simulink model "ExampleWater"  (R2024a)
settings: Solver=FixedStepAuto  StartTime=0.0  StopTime=inf  FixedStep=0.02  RelTol=1e-3  EnableMultiTasking=on
undefined symbols (not defined in the file): atmosphericScattering, basicProperties, bloomBrightnessThreshold, bloomStrength, color, cosInnerCutOffAngle, cosOuterCutOffAngle, direction, emissionColorMultiplier, invRadiusPow4, meshID, pointLightID, position, quadraticFalloff, quaternion, reflectionColorMultiplier, refractionColorMultiplier, scale, shadowBiasMax, shadowBiasMin, shininess, specularColor, spotLightID, strengthDuDvNormal1, strengthDuDvNormal2, textureCoordinateAnimation1, textureCoordinateAnimation2, textureCoordinateScaling1, textureCoordinateScaling2, updateMesh, visible
libraries: PRISMA x49, GenericTarget x2, simulink_extras x1
settings Model: Creator=damerius  LastModifiedBy=Scythe
settings SolverCC: ConcurrentTasks=on  AlgebraicLoopSolver=TrustRegion  PositivePriorityOrder=on
settings DataIOCC: SaveOutput=off  SignalLogging=off  DSMLogging=off  SaveTime=off  ReturnWorkspaceOutputs=off
settings OptimizationCC: DefaultParameterBehavior=Inlined  ReuseModelBlockBuffer=off  ZeroExternalMemoryAtStartup=off  ZeroInternalMemoryAtStartup=off  SimCompilerOptimization=on
settings DebuggingCC: UnconnectedInputMsg=warning  UnconnectedOutputMsg=warning  UnconnectedLineMsg=warning
settings HardwareCC: ProdBitPerLong=64  ProdHWDeviceType=Intel->x86-64 (Linux 64)
settings ModelReferenceCC: EnableRefExpFcnMdlSchedulingChecks=on
settings SFSimCC: SimParseCustomCode=off  SimGenImportedTypeDefs=on  SimTargetLang=C++
settings RTWCC: GenCodeOnly=on  PackageGeneratedCodeAndArtifacts=on  PackageName=PackNGo  RTWVerbose=off  BuildConfiguration=Faster Runs  TargetLang=C++  GPUComputeCapability=3.5  DLArmComputeVersion=19.05
settings CodeAppCC: ForceParamTrailComments=on  MaxIdLength=95  MATLABSourceComments=on  UseSimReservedNames=on
settings GRTTargetCC: TargetLangStandard=C++11 (ISO)  GenerateFullHeader=off  MatFileLogging=off  CodeInterfacePackaging=C++ class

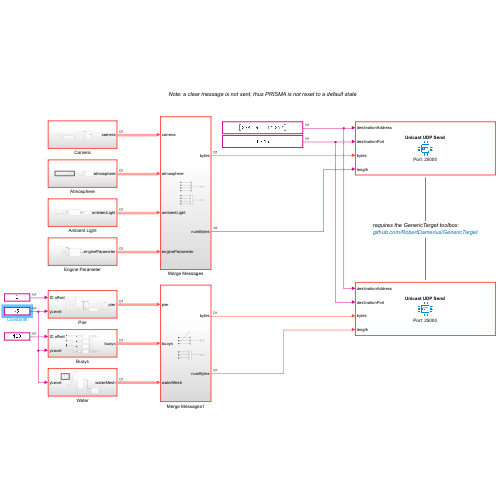
[thumbnail: Simulink's stored preview of the top-level diagram]
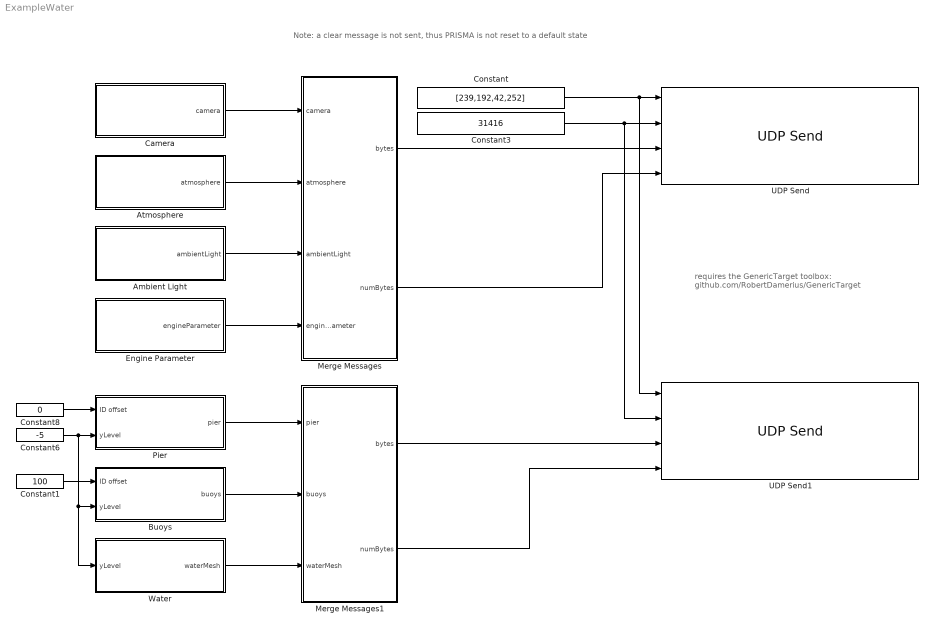
== system ExampleWater ==
  note: Note: a clear message is not sent, thus PRISMA is not reset to a default state
  note: requires the GenericTarget toolbox:
      | github.com/RobertDamerius/GenericTarget
  Ambient Light : Subsystem
  Atmosphere : Subsystem
  Buoys : Subsystem
  Camera : Subsystem
  Constant : Constant  Value=[239,192,42,252]  OutDataTypeStr=uint8
  Constant1 : Constant  Value=100  OutDataTypeStr=uint32
  Constant3 : Constant  Value=31416  OutDataTypeStr=uint16
  Constant6 : Constant  Value=-5
  Constant8 : Constant  Value=0  OutDataTypeStr=uint32
  Engine Parameter : Subsystem
  Merge Messages : Subsystem
  Merge Messages1 : Subsystem
  Pier : Subsystem
  UDP Send : GenericTarget/Interface/UDP Send  showDetails=off  interfacePort=25000  interfaceIP=[0,0,0,0]  deviceName=''  prioritySocket=6  allowBroadcast=off  SampleTime=-1
      settings: SourceProductName=Generic Target
  UDP Send1 : GenericTarget/Interface/UDP Send  showDetails=off  interfacePort=25000  interfaceIP=[0,0,0,0]  deviceName=''  prioritySocket=6  allowBroadcast=off  SampleTime=-1
      settings: SourceProductName=Generic Target
  Water : Subsystem
  wires:
  Constant3/1 -> UDP Send1/2, UDP Send/2
  Camera/1(camera) -> Merge Messages/1(camera)
  Merge Messages/1(bytes) -> UDP Send/3
  Merge Messages/2(numBytes) -> UDP Send/4
  Ambient Light/1(ambientLight) -> Merge Messages/3(ambientLight)
  Constant/1 -> UDP Send1/1, UDP Send/1
  Atmosphere/1(atmosphere) -> Merge Messages/2(atmosphere)
  Engine Parameter/1(engineParameter) -> Merge Messages/4(engineParameter)
  Constant8/1 -> Pier/1(ID offset)
  Constant1/1 -> Buoys/1(ID offset)
  Constant6/1 -> Water/1(yLevel), Buoys/2(yLevel), Pier/2(yLevel)
  Pier/1(pier) -> Merge Messages1/1(pier)
  Buoys/1(buoys) -> Merge Messages1/2(buoys)
  Water/1(waterMesh) -> Merge Messages1/3(waterMesh)
  Merge Messages1/1(bytes) -> UDP Send1/3
  Merge Messages1/2(numBytes) -> UDP Send1/4

== system ExampleWater/Ambient Light ==
  Bus Assignment2 : BusAssignment  AssignedSignals=color
  Constant12 : Constant  Value=[1;1;1]
  Default Ambient Light Bus : PRISMA/Default Ambient Light Bus
      settings: SourceProductName=PRISMA
  Gain : Gain  Gain=0.02
  Pack Ambient Light Message : PRISMA/Pack Ambient Light Message
      settings: SourceProductName=PRISMA
  Bus Element Out : Outport  PortName=ambientLight  Element=bytes
  Bus Element Out1 : Outport  PortName=ambientLight  Element=numBytes
  wires:
  Pack Ambient Light Message/2 -> Bus Element Out1/1
  Pack Ambient Light Message/1 -> Bus Element Out/1
  Gain/1 -> Bus Assignment2/2
  Constant12/1 -> Gain/1
  Default Ambient Light Bus/1 -> Bus Assignment2/1
  Bus Assignment2/1 -> Pack Ambient Light Message/1

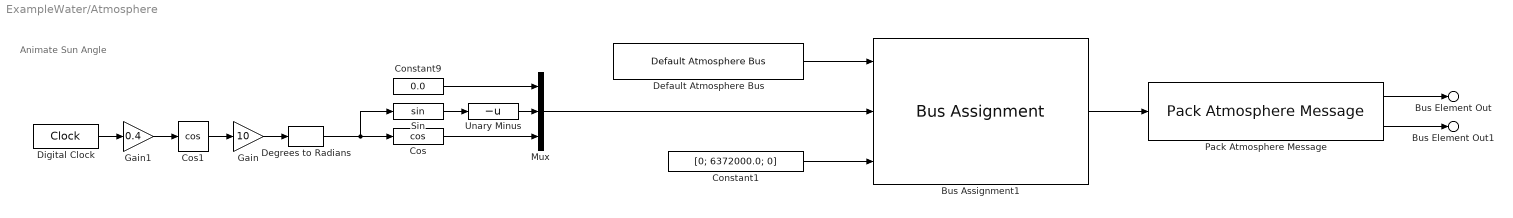
== system ExampleWater/Atmosphere ==
  note: Animate Sun Angle
  Bus Assignment1 : BusAssignment  AssignedSignals=basicProperties.sunLightDirection,atmosphericScattering.eyePosition
  Constant1 : Constant  Value=[0; 6372000.0; 0]
  Constant9 : Constant  Value=0.0
  Cos : Trigonometry  Operator=cos
  Cos1 : Trigonometry  Operator=cos
  Default Atmosphere Bus : PRISMA/Default Atmosphere Bus
      settings: SourceProductName=PRISMA
  Degrees to Radians : simulink_extras/Transformations/Degrees to Radians
  Digital Clock : DigitalClock  SampleTime=0.02
  Gain : Gain  Gain=10
  Gain1 : Gain  Gain=0.4
  Mux : Mux  Inputs=3
  Pack Atmosphere Message : PRISMA/Pack Atmosphere Message
      settings: SourceProductName=PRISMA
  Sin : Trigonometry
  Unary Minus : UnaryMinus
  Bus Element Out : Outport  PortName=atmosphere  Element=bytes
  Bus Element Out1 : Outport  PortName=atmosphere  Element=numBytes
  wires:
  Bus Assignment1/1 -> Pack Atmosphere Message/1
  Default Atmosphere Bus/1 -> Bus Assignment1/1
  Pack Atmosphere Message/1 -> Bus Element Out/1
  Pack Atmosphere Message/2 -> Bus Element Out1/1
  Mux/1 -> Bus Assignment1/2
  Constant1/1 -> Bus Assignment1/3
  Sin/1 -> Unary Minus/1
  Constant9/1 -> Mux/1
  Unary Minus/1 -> Mux/2
  Degrees to Radians/1 -> Sin/1, Cos/1
  Cos/1 -> Mux/3
  Cos1/1 -> Gain/1
  Digital Clock/1 -> Gain1/1
  Gain/1 -> Degrees to Radians/1
  Gain1/1 -> Cos1/1

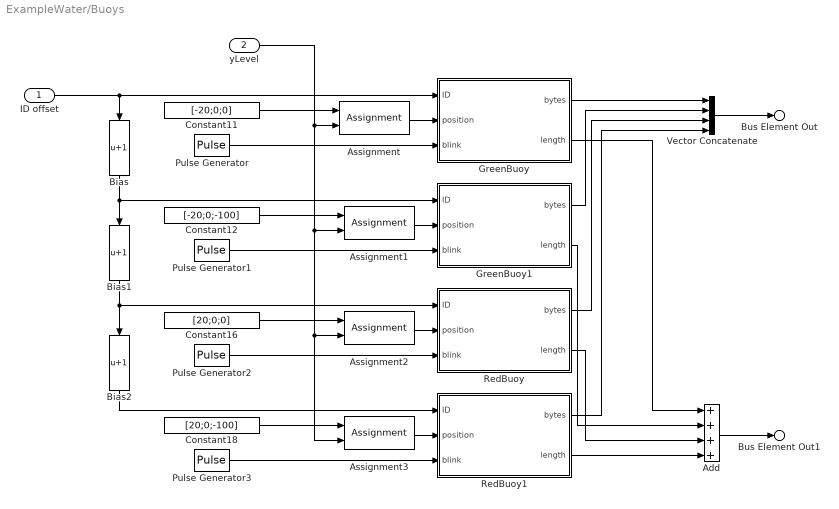
== system ExampleWater/Buoys ==
  ID offset : Inport
  yLevel : Inport  Port=2
  Add : Sum  Inputs=++++
  Assignment{,1..3} (4 alike) : Assignment  DiagnosticForDimensions=Warning  IndexOptions=Index vector (dialog)  Indices=2  OutputSizes=1
  Bias : Bias  Bias=1  SaturateOnIntegerOverflow=off
  Bias1 : Bias  Bias=1  SaturateOnIntegerOverflow=off
  Bias2 : Bias  Bias=1  SaturateOnIntegerOverflow=off
  Constant11 : Constant  Value=[-20;0;0]
  Constant12 : Constant  Value=[-20;0;-100]
  Constant16 : Constant  Value=[20;0;0]
  Constant18 : Constant  Value=[20;0;-100]
  GreenBuoy : Subsystem
  GreenBuoy1 : Subsystem
  Pulse Generator : DiscretePulseGenerator  PulseType=Time based  Period=4  PulseWidth=40
  Pulse Generator1 : DiscretePulseGenerator  PulseType=Time based  Period=5  PulseWidth=60  PhaseDelay=0.9
  Pulse Generator2 : DiscretePulseGenerator  PulseType=Time based  PulseWidth=50  PhaseDelay=1.6
  Pulse Generator3 : DiscretePulseGenerator  PulseType=Time based  Period=3  PulseWidth=30  PhaseDelay=2.8
  RedBuoy : Subsystem
  RedBuoy1 : Subsystem
  Vector Concatenate : Concatenate  NumInputs=4
  Bus Element Out : Outport  PortName=buoys  Element=bytes
  Bus Element Out1 : Outport  PortName=buoys  Element=numBytes
  wires:
  yLevel/1 -> Assignment3/2, Assignment2/2, Assignment1/2, Assignment/2
  Constant18/1 -> Assignment3/1
  Constant16/1 -> Assignment2/1
  Constant12/1 -> Assignment1/1
  Assignment3/1 -> RedBuoy1/2(position)
  Assignment2/1 -> RedBuoy/2(position)
  Assignment1/1 -> GreenBuoy1/2(position)
  Assignment/1 -> GreenBuoy/2(position)
  Pulse Generator3/1 -> RedBuoy1/3(blink)
  Pulse Generator2/1 -> RedBuoy/3(blink)
  Pulse Generator1/1 -> GreenBuoy1/3(blink)
  Pulse Generator/1 -> GreenBuoy/3(blink)
  GreenBuoy/2(length) -> Add/1
  GreenBuoy1/2(length) -> Add/2
  RedBuoy/2(length) -> Add/3
  Constant11/1 -> Assignment/1
  GreenBuoy/1(bytes) -> Vector Concatenate/1
  ID offset/1 -> GreenBuoy/1(ID), Bias/1
  RedBuoy1/1(bytes) -> Vector Concatenate/4
  RedBuoy1/2(length) -> Add/4
  Bias2/1 -> RedBuoy1/1(ID)
  Bias1/1 -> Bias2/1, RedBuoy/1(ID)
  RedBuoy/1(bytes) -> Vector Concatenate/3
  GreenBuoy1/1(bytes) -> Vector Concatenate/2
  Bias/1 -> Bias1/1, GreenBuoy1/1(ID)
  Vector Concatenate/1 -> Bus Element Out/1
  Add/1 -> Bus Element Out1/1

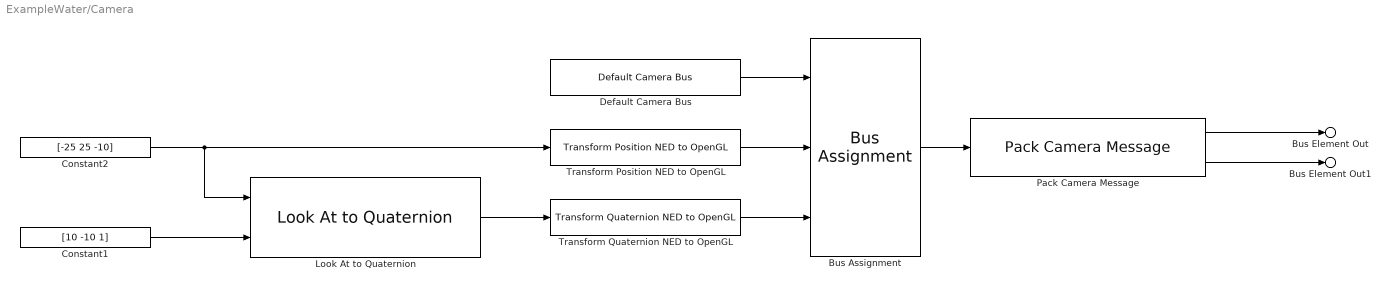
== system ExampleWater/Camera ==
  Bus Assignment : BusAssignment  AssignedSignals=position,quaternion
  Constant1 : Constant  Value=[10 -10 1]
  Constant2 : Constant  Value=[-25 25 -10]
  Default Camera Bus : PRISMA/Default Camera Bus
      settings: SourceProductName=PRISMA
  Look At to Quaternion : PRISMA/Transformation/Look At to Quaternion
      settings: SourceProductName=PRISMA
  Pack Camera Message : PRISMA/Pack Camera Message
      settings: SourceProductName=PRISMA
  Transform Position NED to OpenGL : PRISMA/Transformation/Transform Position NED to OpenGL
      settings: SourceProductName=PRISMA
  Transform Quaternion NED to OpenGL : PRISMA/Transformation/Transform Quaternion NED to OpenGL
      settings: SourceProductName=PRISMA
  Bus Element Out : Outport  PortName=camera  Element=bytes
  Bus Element Out1 : Outport  PortName=camera  Element=numBytes
  wires:
  Default Camera Bus/1 -> Bus Assignment/1
  Bus Assignment/1 -> Pack Camera Message/1
  Transform Position NED to OpenGL/1 -> Bus Assignment/2
  Transform Quaternion NED to OpenGL/1 -> Bus Assignment/3
  Look At to Quaternion/1 -> Transform Quaternion NED to OpenGL/1
  Constant1/1 -> Look At to Quaternion/2
  Pack Camera Message/1 -> Bus Element Out/1
  Pack Camera Message/2 -> Bus Element Out1/1
  Constant2/1 -> Look At to Quaternion/1, Transform Position NED to OpenGL/1

== system ExampleWater/Engine Parameter ==
  Bus Assignment3 : BusAssignment  AssignedSignals=bloomBrightnessThreshold,bloomStrength,shadowBiasMin,shadowBiasMax
  Constant13 : Constant  Value=0
  Constant14 : Constant  Value=0
  Constant2 : Constant
  Constant3 : Constant  Value=0.1
  Default Engine Parameter Bus : PRISMA/Default Engine Parameter Bus
      settings: SourceProductName=PRISMA
  Pack Engine Parameter Message : PRISMA/Pack Engine Parameter Message
      settings: SourceProductName=PRISMA
  Bus Element Out : Outport  PortName=engineParameter  Element=bytes
  Bus Element Out1 : Outport  PortName=engineParameter  Element=numBytes
  wires:
  Pack Engine Parameter Message/1 -> Bus Element Out/1
  Pack Engine Parameter Message/2 -> Bus Element Out1/1
  Constant14/1 -> Bus Assignment3/5
  Constant13/1 -> Bus Assignment3/4
  Constant3/1 -> Bus Assignment3/3
  Constant2/1 -> Bus Assignment3/2
  Default Engine Parameter Bus/1 -> Bus Assignment3/1
  Bus Assignment3/1 -> Pack Engine Parameter Message/1

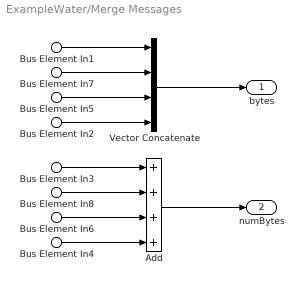
== system ExampleWater/Merge Messages ==
  Bus Element In1 : Inport  PortName=camera  Element=bytes
  Bus Element In3 : Inport  PortName=camera  Element=numBytes
  Bus Element In7 : Inport  Port=2  PortName=atmosphere  Element=bytes
  Bus Element In8 : Inport  Port=2  PortName=atmosphere  Element=numBytes
  Bus Element In5 : Inport  Port=3  PortName=ambientLight  Element=bytes
  Bus Element In6 : Inport  Port=3  PortName=ambientLight  Element=numBytes
  Bus Element In2 : Inport  Port=4  PortName=engineParameter  Element=bytes
  Bus Element In4 : Inport  Port=4  PortName=engineParameter  Element=numBytes
  Add : Sum  Inputs=++++
  Vector Concatenate : Concatenate  NumInputs=4
  bytes : Outport
  numBytes : Outport  Port=2
  wires:
  Bus Element In1/1 -> Vector Concatenate/1
  Bus Element In2/1 -> Vector Concatenate/4
  Bus Element In3/1 -> Add/1
  Bus Element In4/1 -> Add/4
  Vector Concatenate/1 -> bytes/1
  Add/1 -> numBytes/1
  Bus Element In5/1 -> Vector Concatenate/3
  Bus Element In6/1 -> Add/3
  Bus Element In7/1 -> Vector Concatenate/2
  Bus Element In8/1 -> Add/2

== system ExampleWater/Merge Messages1 ==
  note: water mesh has a fixed size for variable length data:
      | use it as last value for merging
  Bus Element In1 : Inport  PortName=pier  Element=bytes
  Bus Element In3 : Inport  PortName=pier  Element=numBytes
  Bus Element In7 : Inport  Port=2  PortName=buoys  Element=bytes
  Bus Element In8 : Inport  Port=2  PortName=buoys  Element=numBytes
  Bus Element In5 : Inport  Port=3  PortName=waterMesh  Element=bytes
  Bus Element In6 : Inport  Port=3  PortName=waterMesh  Element=numBytes
  Add : Sum  Inputs=+++
  Vector Concatenate : Concatenate  NumInputs=3
  bytes : Outport
  numBytes : Outport  Port=2
  wires:
  Bus Element In8/1 -> Add/2
  Bus Element In7/1 -> Vector Concatenate/2
  Bus Element In6/1 -> Add/3
  Bus Element In5/1 -> Vector Concatenate/3
  Add/1 -> numBytes/1
  Vector Concatenate/1 -> bytes/1
  Bus Element In3/1 -> Add/1
  Bus Element In1/1 -> Vector Concatenate/1

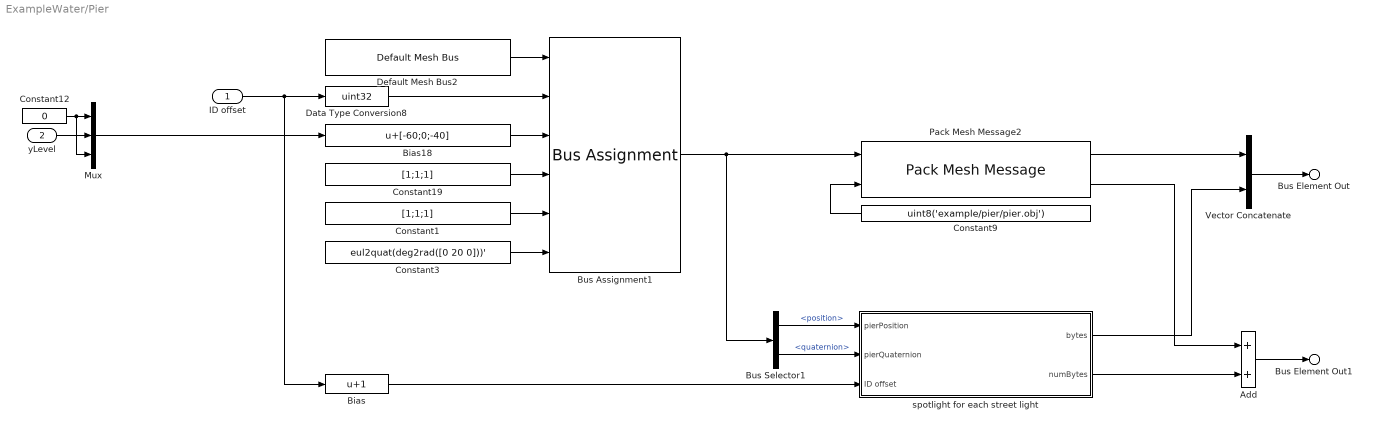
== system ExampleWater/Pier ==
  ID offset : Inport
  yLevel : Inport  Port=2
  Add : Sum
  Bias : Bias  Bias=1  SaturateOnIntegerOverflow=off
  Bias18 : Bias  Bias=[-60;0;-40]  SaturateOnIntegerOverflow=off
  Bus Assignment1 : BusAssignment  AssignedSignals=meshID,position,scale,emissionColorMultiplier,quaternion
  Bus Selector1 : BusSelector  OutputSignals=position,quaternion
  Constant1 : Constant  Value=[1;1;1]
  Constant12 : Constant  Value=0
  Constant19 : Constant  Value=[1;1;1]
  Constant3 : Constant  Value=eul2quat(deg2rad([0 20 0]))'
  Constant9 : Constant  Value=uint8('example/pier/pier.obj')  OutDataTypeStr=uint8
  Data Type Conversion8 : DataTypeConversion  OutDataTypeStr=uint32  SaturateOnIntegerOverflow=off  RndMeth=Floor
  Default Mesh Bus2 : PRISMA/Default Mesh Bus
      settings: SourceProductName=PRISMA
  Mux : Mux  Inputs=3
  Pack Mesh Message2 : PRISMA/Pack Mesh Message
      settings: SourceProductName=PRISMA
  Vector Concatenate : Concatenate
  spotlight for each street light : Subsystem
  Bus Element Out : Outport  PortName=pier  Element=bytes
  Bus Element Out1 : Outport  PortName=pier  Element=numBytes
  wires:
  Constant3/1 -> Bus Assignment1/6
  Pack Mesh Message2/2 -> Add/1
  Constant1/1 -> Bus Assignment1/5
  Constant9/1 -> Pack Mesh Message2/2
  Default Mesh Bus2/1 -> Bus Assignment1/1
  Constant19/1 -> Bus Assignment1/4
  Bus Assignment1/1 -> Bus Selector1/1, Pack Mesh Message2/1
  Data Type Conversion8/1 -> Bus Assignment1/2
  Mux/1 -> Bias18/1
  Pack Mesh Message2/1 -> Vector Concatenate/1
  ID offset/1 -> Bias/1, Data Type Conversion8/1
  Constant12/1 -> Mux/3, Mux/1
  yLevel/1 -> Mux/2
  Bias18/1 -> Bus Assignment1/3
  spotlight for each street light/1(bytes) -> Vector Concatenate/2
  spotlight for each street light/2(numBytes) -> Add/2
  Bias/1 -> spotlight for each street light/3(ID offset)
  Bus Selector1/1 -> spotlight for each street light/1(pierPosition)  "<position>"
  Bus Selector1/2 -> spotlight for each street light/2(pierQuaternion)  "<quaternion>"
  Vector Concatenate/1 -> Bus Element Out/1
  Add/1 -> Bus Element Out1/1

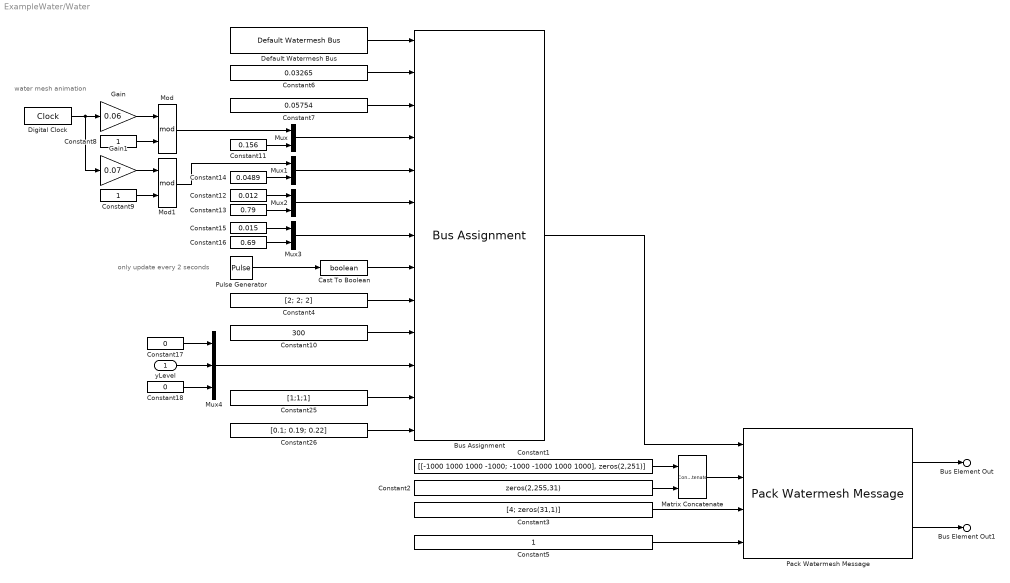
== system ExampleWater/Water ==
  note: only update every 2 seconds
  note: water mesh animation
  yLevel : Inport
  Bus Assignment : BusAssignment  AssignedSignals=textureCoordinateScaling1,textureCoordinateScaling2,textureCoordinateAnimation1,textureCoordinateAnimation2,strengthDuDvNormal1,strengthDuDvNormal2,updateMesh,specularColor,shininess,position,reflectionColorMultiplier,refractionColorMultiplier
  Cast To Boolean : DataTypeConversion  OutDataTypeStr=boolean  SaturateOnIntegerOverflow=off  RndMeth=Floor
  Constant1 : Constant  Value=[[-1000 1000 1000 -1000; -1000 -1000 1000 1000], zeros(2,251)]
  Constant10 : Constant  Value=300
  Constant11 : Constant  Value=0.156
  Constant12 : Constant  Value=0.012
  Constant13 : Constant  Value=0.79
  Constant14 : Constant  Value=0.0489
  Constant15 : Constant  Value=0.015
  Constant16 : Constant  Value=0.69
  Constant17 : Constant  Value=0
  Constant18 : Constant  Value=0
  Constant2 : Constant  Value=zeros(2,255,31)
  Constant25 : Constant  Value=[1;1;1]
  Constant26 : Constant  Value=[0.1; 0.19; 0.22]
  Constant3 : Constant  Value=[4; zeros(31,1)]  OutDataTypeStr=uint8
  Constant4 : Constant  Value=[2; 2; 2]
  Constant5 : Constant  OutDataTypeStr=uint8
  Constant6 : Constant  Value=0.03265
  Constant7 : Constant  Value=0.05754
  Constant8 : Constant
  Constant9 : Constant
  Default Watermesh Bus : PRISMA/Default Watermesh Bus
      settings: SourceProductName=PRISMA
  Digital Clock : DigitalClock  SampleTime=0.02
  Gain : Gain  Gain=0.06
  Gain1 : Gain  Gain=0.07
  Matrix Concatenate : Concatenate  Mode=Multidimensional array  ConcatenateDimension=3
  Mod : Math  Operator=mod
  Mod1 : Math  Operator=mod
  Mux{,1..3} (4 alike) : Mux  Inputs=2
  Mux4 : Mux  Inputs=3
  Pack Watermesh Message : PRISMA/Pack Watermesh Message
      settings: SourceProductName=PRISMA
  Pulse Generator : DiscretePulseGenerator  Period=100  SampleTime=0.02
  Bus Element Out : Outport  PortName=waterMesh  Element=bytes
  Bus Element Out1 : Outport  PortName=waterMesh  Element=numBytes
  wires:
  Constant25/1 -> Bus Assignment/12
  Constant26/1 -> Bus Assignment/13
  Mux2/1 -> Bus Assignment/6
  Constant18/1 -> Mux4/3
  yLevel/1 -> Mux4/2
  Constant17/1 -> Mux4/1
  Mux4/1 -> Bus Assignment/11
  Constant10/1 -> Bus Assignment/10
  Gain1/1 -> Mod1/1
  Mod/1 -> Mux/1
  Constant13/1 -> Mux2/2
  Constant8/1 -> Mod/2
  Mux3/1 -> Bus Assignment/7
  Constant14/1 -> Mux1/2
  Constant6/1 -> Bus Assignment/2
  Mux1/1 -> Bus Assignment/5
  Default Watermesh Bus/1 -> Bus Assignment/1
  Constant12/1 -> Mux2/1
  Constant16/1 -> Mux3/2
  Constant9/1 -> Mod1/2
  Constant15/1 -> Mux3/1
  Pulse Generator/1 -> Cast To Boolean/1
  Mod1/1 -> Mux1/1
  Constant5/1 -> Pack Watermesh Message/4
  Mux/1 -> Bus Assignment/4
  Constant3/1 -> Pack Watermesh Message/3
  Matrix Concatenate/1 -> Pack Watermesh Message/2
  Constant7/1 -> Bus Assignment/3
  Constant2/1 -> Matrix Concatenate/2
  Bus Assignment/1 -> Pack Watermesh Message/1
  Constant1/1 -> Matrix Concatenate/1
  Constant11/1 -> Mux/2
  Gain/1 -> Mod/1
  Cast To Boolean/1 -> Bus Assignment/8
  Digital Clock/1 -> Gain/1, Gain1/1
  Pack Watermesh Message/1 -> Bus Element Out/1
  Pack Watermesh Message/2 -> Bus Element Out1/1
  Constant4/1 -> Bus Assignment/9

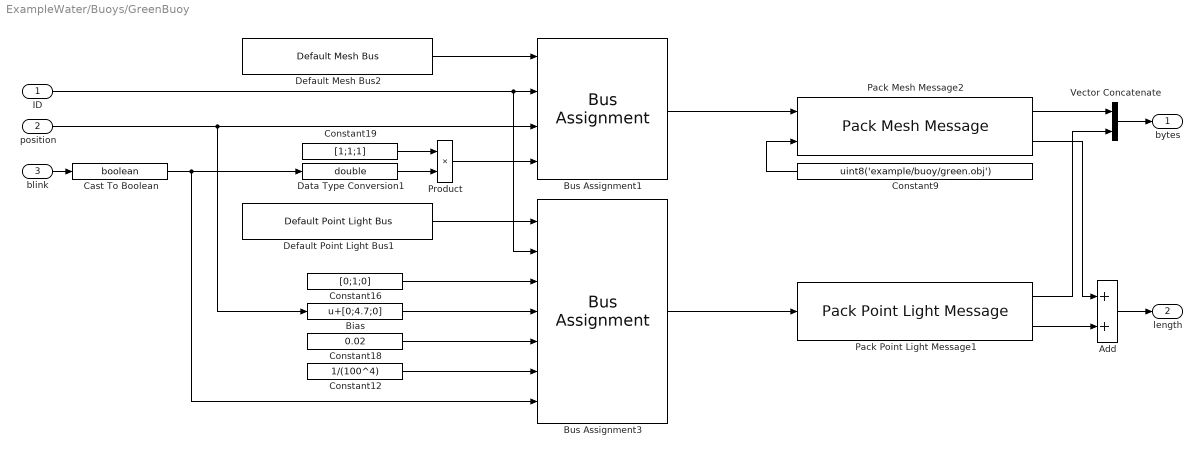
== system ExampleWater/Buoys/GreenBuoy ==
  ID : Inport
  position : Inport  Port=2
  blink : Inport  Port=3
  Add : Sum
  Bias : Bias  Bias=[0;4.7;0]  SaturateOnIntegerOverflow=off
  Bus Assignment1 : BusAssignment  AssignedSignals=meshID,position,emissionColorMultiplier
  Bus Assignment3 : BusAssignment  AssignedSignals=pointLightID,color,position,quadraticFalloff,invRadiusPow4,visible
  Cast To Boolean : DataTypeConversion  OutDataTypeStr=boolean  SaturateOnIntegerOverflow=off  RndMeth=Floor
  Constant12 : Constant  Value=1/(100^4)
  Constant16 : Constant  Value=[0;1;0]
  Constant18 : Constant  Value=0.02
  Constant19 : Constant  Value=[1;1;1]
  Constant9 : Constant  Value=uint8('example/buoy/green.obj')  OutDataTypeStr=uint8
  Data Type Conversion1 : DataTypeConversion  OutDataTypeStr=double  SaturateOnIntegerOverflow=off  RndMeth=Floor
  Default Mesh Bus2 : PRISMA/Default Mesh Bus
      settings: SourceProductName=PRISMA
  Default Point Light Bus1 : PRISMA/Default Point Light Bus
      settings: SourceProductName=PRISMA
  Pack Mesh Message2 : PRISMA/Pack Mesh Message
      settings: SourceProductName=PRISMA
  Pack Point Light Message1 : PRISMA/Pack Point Light Message
      settings: SourceProductName=PRISMA
  Product : Product
  Vector Concatenate : Concatenate
  bytes : Outport
  length : Outport  Port=2
  wires:
  ID/1 -> Bus Assignment1/2, Bus Assignment3/2
  Constant12/1 -> Bus Assignment3/6
  Constant18/1 -> Bus Assignment3/5
  Bias/1 -> Bus Assignment3/4
  Constant16/1 -> Bus Assignment3/3
  Product/1 -> Bus Assignment1/4
  position/1 -> Bias/1, Bus Assignment1/3
  blink/1 -> Cast To Boolean/1
  Vector Concatenate/1 -> bytes/1
  Pack Mesh Message2/2 -> Add/1
  Bus Assignment3/1 -> Pack Point Light Message1/1
  Add/1 -> length/1
  Constant9/1 -> Pack Mesh Message2/2
  Pack Point Light Message1/1 -> Vector Concatenate/2
  Pack Point Light Message1/2 -> Add/2
  Bus Assignment1/1 -> Pack Mesh Message2/1
  Constant19/1 -> Product/1
  Pack Mesh Message2/1 -> Vector Concatenate/1
  Default Point Light Bus1/1 -> Bus Assignment3/1
  Cast To Boolean/1 -> Bus Assignment3/7, Data Type Conversion1/1
  Data Type Conversion1/1 -> Product/2
  Default Mesh Bus2/1 -> Bus Assignment1/1

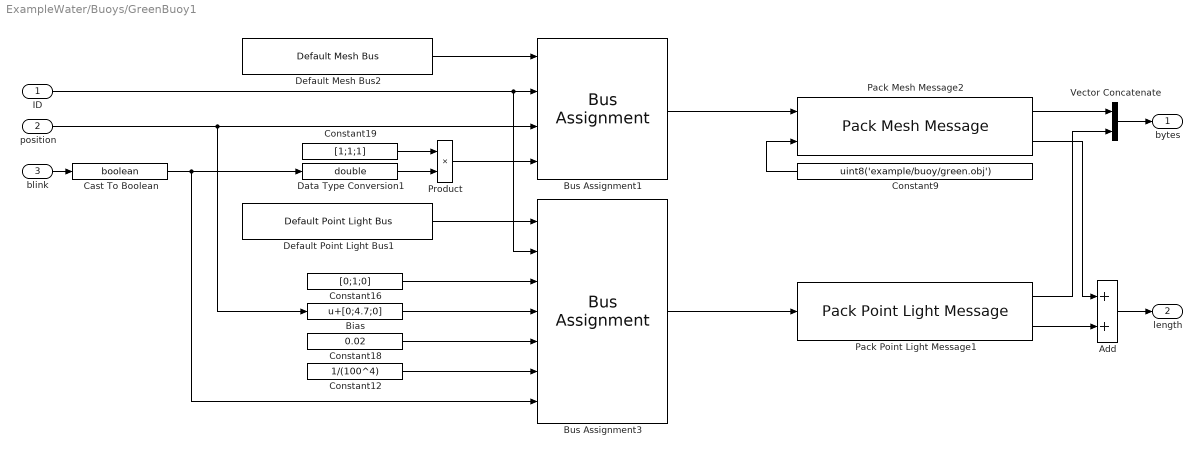
== system ExampleWater/Buoys/GreenBuoy1 ==
  ID : Inport
  position : Inport  Port=2
  blink : Inport  Port=3
  Add : Sum
  Bias : Bias  Bias=[0;4.7;0]  SaturateOnIntegerOverflow=off
  Bus Assignment1 : BusAssignment  AssignedSignals=meshID,position,emissionColorMultiplier
  Bus Assignment3 : BusAssignment  AssignedSignals=pointLightID,color,position,quadraticFalloff,invRadiusPow4,visible
  Cast To Boolean : DataTypeConversion  OutDataTypeStr=boolean  SaturateOnIntegerOverflow=off  RndMeth=Floor
  Constant12 : Constant  Value=1/(100^4)
  Constant16 : Constant  Value=[0;1;0]
  Constant18 : Constant  Value=0.02
  Constant19 : Constant  Value=[1;1;1]
  Constant9 : Constant  Value=uint8('example/buoy/green.obj')  OutDataTypeStr=uint8
  Data Type Conversion1 : DataTypeConversion  OutDataTypeStr=double  SaturateOnIntegerOverflow=off  RndMeth=Floor
  Default Mesh Bus2 : PRISMA/Default Mesh Bus
      settings: SourceProductName=PRISMA
  Default Point Light Bus1 : PRISMA/Default Point Light Bus
      settings: SourceProductName=PRISMA
  Pack Mesh Message2 : PRISMA/Pack Mesh Message
      settings: SourceProductName=PRISMA
  Pack Point Light Message1 : PRISMA/Pack Point Light Message
      settings: SourceProductName=PRISMA
  Product : Product
  Vector Concatenate : Concatenate
  bytes : Outport
  length : Outport  Port=2
  wires:
  Default Mesh Bus2/1 -> Bus Assignment1/1
  Data Type Conversion1/1 -> Product/2
  Cast To Boolean/1 -> Data Type Conversion1/1, Bus Assignment3/7
  Default Point Light Bus1/1 -> Bus Assignment3/1
  Pack Mesh Message2/1 -> Vector Concatenate/1
  Constant19/1 -> Product/1
  Bus Assignment1/1 -> Pack Mesh Message2/1
  Pack Point Light Message1/2 -> Add/2
  Pack Point Light Message1/1 -> Vector Concatenate/2
  Constant9/1 -> Pack Mesh Message2/2
  Add/1 -> length/1
  Bus Assignment3/1 -> Pack Point Light Message1/1
  Pack Mesh Message2/2 -> Add/1
  Vector Concatenate/1 -> bytes/1
  blink/1 -> Cast To Boolean/1
  position/1 -> Bias/1, Bus Assignment1/3
  Product/1 -> Bus Assignment1/4
  Constant16/1 -> Bus Assignment3/3
  Bias/1 -> Bus Assignment3/4
  Constant18/1 -> Bus Assignment3/5
  Constant12/1 -> Bus Assignment3/6
  ID/1 -> Bus Assignment3/2, Bus Assignment1/2

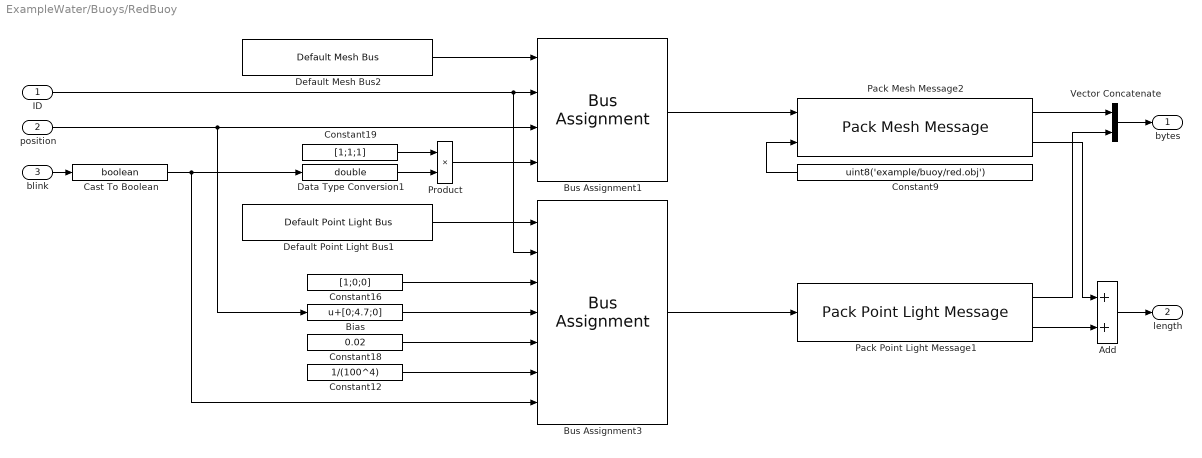
== system ExampleWater/Buoys/RedBuoy ==
  ID : Inport
  position : Inport  Port=2
  blink : Inport  Port=3
  Add : Sum
  Bias : Bias  Bias=[0;4.7;0]  SaturateOnIntegerOverflow=off
  Bus Assignment1 : BusAssignment  AssignedSignals=meshID,position,emissionColorMultiplier
  Bus Assignment3 : BusAssignment  AssignedSignals=pointLightID,color,position,quadraticFalloff,invRadiusPow4,visible
  Cast To Boolean : DataTypeConversion  OutDataTypeStr=boolean  SaturateOnIntegerOverflow=off  RndMeth=Floor
  Constant12 : Constant  Value=1/(100^4)
  Constant16 : Constant  Value=[1;0;0]
  Constant18 : Constant  Value=0.02
  Constant19 : Constant  Value=[1;1;1]
  Constant9 : Constant  Value=uint8('example/buoy/red.obj')  OutDataTypeStr=uint8
  Data Type Conversion1 : DataTypeConversion  OutDataTypeStr=double  SaturateOnIntegerOverflow=off  RndMeth=Floor
  Default Mesh Bus2 : PRISMA/Default Mesh Bus
      settings: SourceProductName=PRISMA
  Default Point Light Bus1 : PRISMA/Default Point Light Bus
      settings: SourceProductName=PRISMA
  Pack Mesh Message2 : PRISMA/Pack Mesh Message
      settings: SourceProductName=PRISMA
  Pack Point Light Message1 : PRISMA/Pack Point Light Message
      settings: SourceProductName=PRISMA
  Product : Product
  Vector Concatenate : Concatenate
  bytes : Outport
  length : Outport  Port=2
  wires:
  ID/1 -> Bus Assignment1/2, Bus Assignment3/2
  Constant12/1 -> Bus Assignment3/6
  Constant18/1 -> Bus Assignment3/5
  Bias/1 -> Bus Assignment3/4
  Constant16/1 -> Bus Assignment3/3
  Product/1 -> Bus Assignment1/4
  position/1 -> Bias/1, Bus Assignment1/3
  blink/1 -> Cast To Boolean/1
  Vector Concatenate/1 -> bytes/1
  Pack Mesh Message2/2 -> Add/1
  Bus Assignment3/1 -> Pack Point Light Message1/1
  Add/1 -> length/1
  Constant9/1 -> Pack Mesh Message2/2
  Pack Point Light Message1/1 -> Vector Concatenate/2
  Pack Point Light Message1/2 -> Add/2
  Bus Assignment1/1 -> Pack Mesh Message2/1
  Constant19/1 -> Product/1
  Pack Mesh Message2/1 -> Vector Concatenate/1
  Default Point Light Bus1/1 -> Bus Assignment3/1
  Cast To Boolean/1 -> Bus Assignment3/7, Data Type Conversion1/1
  Data Type Conversion1/1 -> Product/2
  Default Mesh Bus2/1 -> Bus Assignment1/1

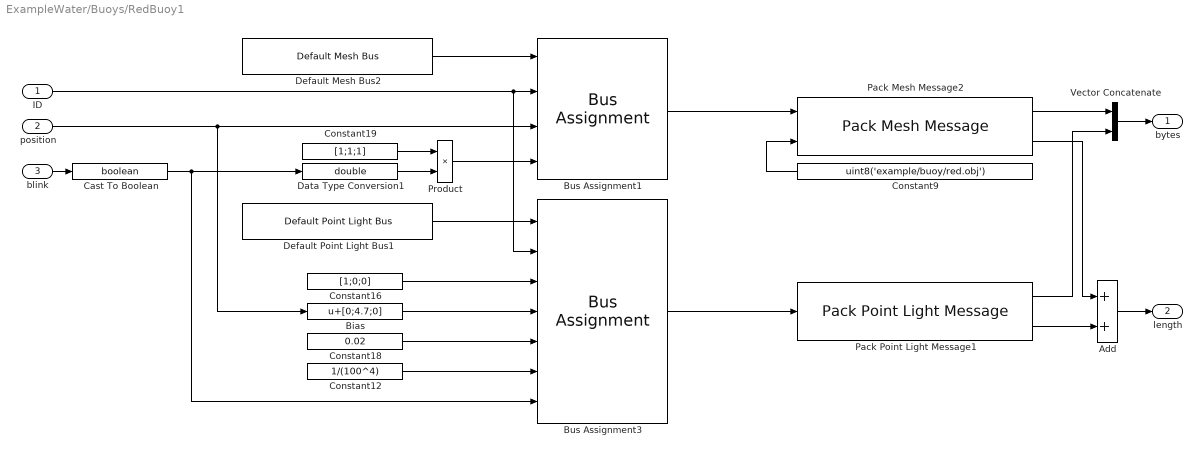
== system ExampleWater/Buoys/RedBuoy1 ==
  ID : Inport
  position : Inport  Port=2
  blink : Inport  Port=3
  Add : Sum
  Bias : Bias  Bias=[0;4.7;0]  SaturateOnIntegerOverflow=off
  Bus Assignment1 : BusAssignment  AssignedSignals=meshID,position,emissionColorMultiplier
  Bus Assignment3 : BusAssignment  AssignedSignals=pointLightID,color,position,quadraticFalloff,invRadiusPow4,visible
  Cast To Boolean : DataTypeConversion  OutDataTypeStr=boolean  SaturateOnIntegerOverflow=off  RndMeth=Floor
  Constant12 : Constant  Value=1/(100^4)
  Constant16 : Constant  Value=[1;0;0]
  Constant18 : Constant  Value=0.02
  Constant19 : Constant  Value=[1;1;1]
  Constant9 : Constant  Value=uint8('example/buoy/red.obj')  OutDataTypeStr=uint8
  Data Type Conversion1 : DataTypeConversion  OutDataTypeStr=double  SaturateOnIntegerOverflow=off  RndMeth=Floor
  Default Mesh Bus2 : PRISMA/Default Mesh Bus
      settings: SourceProductName=PRISMA
  Default Point Light Bus1 : PRISMA/Default Point Light Bus
      settings: SourceProductName=PRISMA
  Pack Mesh Message2 : PRISMA/Pack Mesh Message
      settings: SourceProductName=PRISMA
  Pack Point Light Message1 : PRISMA/Pack Point Light Message
      settings: SourceProductName=PRISMA
  Product : Product
  Vector Concatenate : Concatenate
  bytes : Outport
  length : Outport  Port=2
  wires:
  Default Mesh Bus2/1 -> Bus Assignment1/1
  Data Type Conversion1/1 -> Product/2
  Cast To Boolean/1 -> Data Type Conversion1/1, Bus Assignment3/7
  Default Point Light Bus1/1 -> Bus Assignment3/1
  Pack Mesh Message2/1 -> Vector Concatenate/1
  Constant19/1 -> Product/1
  Bus Assignment1/1 -> Pack Mesh Message2/1
  Pack Point Light Message1/2 -> Add/2
  Pack Point Light Message1/1 -> Vector Concatenate/2
  Constant9/1 -> Pack Mesh Message2/2
  Add/1 -> length/1
  Bus Assignment3/1 -> Pack Point Light Message1/1
  Pack Mesh Message2/2 -> Add/1
  Vector Concatenate/1 -> bytes/1
  blink/1 -> Cast To Boolean/1
  position/1 -> Bias/1, Bus Assignment1/3
  Product/1 -> Bus Assignment1/4
  Constant16/1 -> Bus Assignment3/3
  Bias/1 -> Bus Assignment3/4
  Constant18/1 -> Bus Assignment3/5
  Constant12/1 -> Bus Assignment3/6
  ID/1 -> Bus Assignment3/2, Bus Assignment1/2

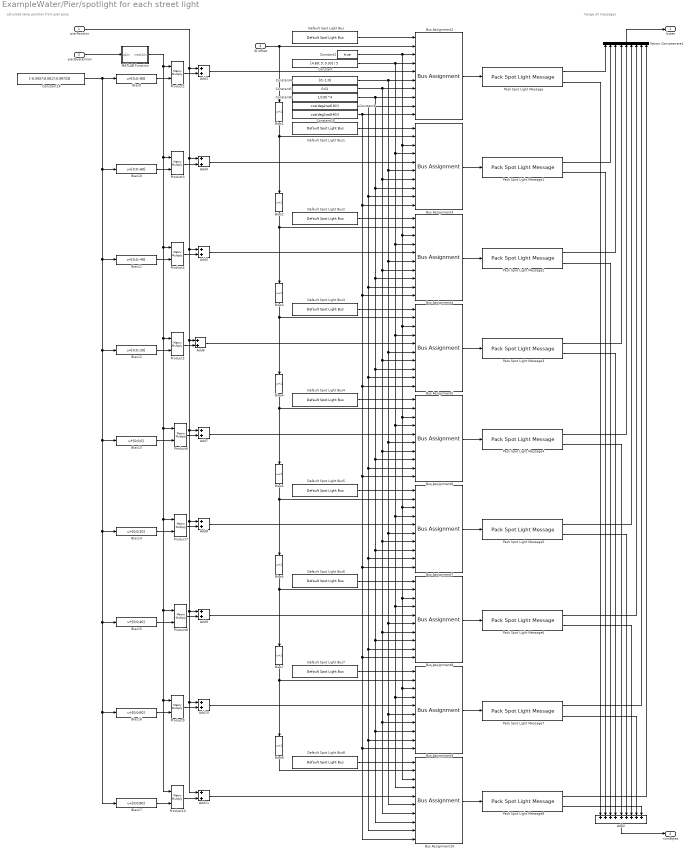
== system ExampleWater/Pier/spotlight for each street light ==
  note: calculate lamp position from pier pose
  note: merge all messages
  pierPosition : Inport
  pierQuaternion : Inport  Port=2
  ID offset : Inport  Port=3
  Add{3..11} (9 alike) : Sum
  Add2 : Sum  Inputs=+++++++++
  Bias{1..8} (8 alike) : Bias  Bias=1  SaturateOnIntegerOverflow=off
  Bias10 : Bias  Bias=[0;0;-60]  SaturateOnIntegerOverflow=off
  Bias11 : Bias  Bias=[0;0;-40]  SaturateOnIntegerOverflow=off
  Bias12 : Bias  Bias=[0;0;-20]  SaturateOnIntegerOverflow=off
  Bias13 : Bias  Bias=[0;0;0]  SaturateOnIntegerOverflow=off
  Bias14 : Bias  Bias=[0;0;20]  SaturateOnIntegerOverflow=off
  Bias15 : Bias  Bias=[0;0;40]  SaturateOnIntegerOverflow=off
  Bias16 : Bias  Bias=[0;0;60]  SaturateOnIntegerOverflow=off
  Bias17 : Bias  Bias=[0;0;80]  SaturateOnIntegerOverflow=off
  Bias9 : Bias  Bias=[0;0;-80]  SaturateOnIntegerOverflow=off
  Bus Assignment{2..10} (9 alike) : BusAssignment  AssignedSignals=spotLightID,visible,color,position,direction,quadraticFalloff,invRadiusPow4,cosInnerCutOffAngle,cosOuterCutOffAngle
  Constant : Constant  Value=[4.69; 5; 3.33] / 5
  Constant10 : Constant  Value=cos(deg2rad(40))
  Constant14 : Constant  Value=[-6.5557;8.0617;0.99725]
  Constant2 : Constant  Value=true  OutDataTypeStr=boolean
  Constant4 : Constant  Value=[0;-1;0]
  Constant5 : Constant  Value=0.01
  Constant6 : Constant  Value=1/(10)^4
  Constant8 : Constant  Value=cos(deg2rad(30))
  Default Spot Light Bus{,1..8} (9 alike) : PRISMA/Default Spot Light Bus
      settings: SourceProductName=PRISMA
  MATLAB Function : MATLAB Function  TreatAsAtomicUnit=on
  Pack Spot Light Message{,1..8} (9 alike) : PRISMA/Pack Spot Light Message
      settings: SourceProductName=PRISMA
  Product{2..10} (9 alike) : Product  Multiplication=Matrix(*)
  Vector Concatenate1 : Concatenate  NumInputs=9
  bytes : Outport
  numBytes : Outport  Port=2
  wires:
  Bias3/1 -> Bias4/1, Bus Assignment5/2
  Product6/1 -> Add7/2
  Pack Spot Light Message5/1 -> Vector Concatenate1/6
  Bias6/1 -> Bias7/1, Bus Assignment8/2
  Product9/1 -> Add10/2
  MATLAB Function/1(matCb2n) -> Product2/1, Product3/1, Product4/1, Product5/1, Product6/1, Product7/1, Product8/1, Product9/1, Product10/1
  Default Spot Light Bus5/1 -> Bus Assignment7/1
  Constant8/1 -> Bus Assignment2/9, Bus Assignment3/9, Bus Assignment4/9, Bus Assignment6/9, Bus Assignment9/9, Bus Assignment10/9, Bus Assignment8/9, Bus Assignment7/9, Bus Assignment5/9
  Constant/1 -> Bus Assignment2/4, Bus Assignment3/4, Bus Assignment4/4, Bus Assignment6/4, Bus Assignment9/4, Bus Assignment10/4, Bus Assignment8/4, Bus Assignment7/4, Bus Assignment5/4
  Add5/1 -> Bus Assignment4/5
  Constant10/1 -> Bus Assignment2/10, Bus Assignment3/10, Bus Assignment4/10, Bus Assignment6/10, Bus Assignment9/10, Bus Assignment10/10, Bus Assignment8/10, Bus Assignment7/10, Bus Assignment5/10
  Constant2/1 -> Bus Assignment2/3, Bus Assignment3/3, Bus Assignment4/3, Bus Assignment6/3, Bus Assignment9/3, Bus Assignment10/3, Bus Assignment8/3, Bus Assignment7/3, Bus Assignment5/3
  Add11/1 -> Bus Assignment10/5
  Pack Spot Light Message4/1 -> Vector Concatenate1/5
  Bias4/1 -> Bus Assignment6/2, Bias5/1
  Product2/1 -> Add3/2
  Pack Spot Light Message6/1 -> Vector Concatenate1/7
  Bias10/1 -> Product3/2
  Constant14/1 -> Bias9/1, Bias17/1, Bias16/1, Bias15/1, Bias14/1, Bias13/1, Bias12/1, Bias11/1, Bias10/1
  ID offset/1 -> Bus Assignment2/2, Bias1/1
  Product3/1 -> Add4/2
  Pack Spot Light Message1/1 -> Vector Concatenate1/2
  Bus Assignment2/1 -> Pack Spot Light Message/1
  Bias8/1 -> Bus Assignment10/2
  Bias1/1 -> Bus Assignment3/2, Bias2/1
  Bias13/1 -> Product6/2
  Default Spot Light Bus1/1 -> Bus Assignment3/1
  Constant4/1 -> Bus Assignment2/6, Bus Assignment3/6, Bus Assignment4/6, Bus Assignment6/6, Bus Assignment9/6, Bus Assignment10/6, Bus Assignment8/6, Bus Assignment7/6, Bus Assignment5/6
  Default Spot Light Bus3/1 -> Bus Assignment5/1
  pierQuaternion/1 -> MATLAB Function/1(qb2n)
  Default Spot Light Bus4/1 -> Bus Assignment6/1
  Bias17/1 -> Product10/2
  Bias11/1 -> Product4/2
  Constant6/1 -> Bus Assignment2/8, Bus Assignment3/8, Bus Assignment4/8, Bus Assignment6/8, Bus Assignment9/8, Bus Assignment10/8, Bus Assignment8/8, Bus Assignment7/8, Bus Assignment5/8
  Add4/1 -> Bus Assignment3/5
  Add3/1 -> Bus Assignment2/5
  Product10/1 -> Add11/2
  Default Spot Light Bus6/1 -> Bus Assignment8/1
  Constant5/1 -> Bus Assignment2/7, Bus Assignment3/7, Bus Assignment4/7, Bus Assignment6/7, Bus Assignment9/7, Bus Assignment10/7, Bus Assignment8/7, Bus Assignment7/7, Bus Assignment5/7
  Bus Assignment4/1 -> Pack Spot Light Message2/1
  Bus Assignment8/1 -> Pack Spot Light Message6/1
  Add9/1 -> Bus Assignment8/5
  Bias2/1 -> Bus Assignment4/2, Bias3/1
  Bus Assignment9/1 -> Pack Spot Light Message7/1
  Add10/1 -> Bus Assignment9/5
  pierPosition/1 -> Add3/1, Add4/1, Add11/1, Add10/1, Add9/1, Add8/1, Add7/1, Add6/1, Add5/1
  Default Spot Light Bus7/1 -> Bus Assignment9/1
  Pack Spot Light Message8/1 -> Vector Concatenate1/9
  Add8/1 -> Bus Assignment7/5
  Add6/1 -> Bus Assignment5/5
  Pack Spot Light Message7/1 -> Vector Concatenate1/8
  Add7/1 -> Bus Assignment6/5
  Product7/1 -> Add8/2
  Product5/1 -> Add6/2
  Bias9/1 -> Product2/2
  Bias16/1 -> Product9/2
  Bias7/1 -> Bus Assignment9/2, Bias8/1
  Bias12/1 -> Product5/2
  Product8/1 -> Add9/2
  Bias5/1 -> Bias6/1, Bus Assignment7/2
  Pack Spot Light Message2/1 -> Vector Concatenate1/3
  Bus Assignment5/1 -> Pack Spot Light Message3/1
  Bus Assignment6/1 -> Pack Spot Light Message4/1
  Bus Assignment7/1 -> Pack Spot Light Message5/1
  Pack Spot Light Message/1 -> Vector Concatenate1/1
  Product4/1 -> Add5/2
  Bus Assignment10/1 -> Pack Spot Light Message8/1
  Default Spot Light Bus8/1 -> Bus Assignment10/1
  Bias14/1 -> Product7/2
  Pack Spot Light Message3/1 -> Vector Concatenate1/4
  Bias15/1 -> Product8/2
  Add2/1 -> numBytes/1
  Default Spot Light Bus2/1 -> Bus Assignment4/1
  Bus Assignment3/1 -> Pack Spot Light Message1/1
  Default Spot Light Bus/1 -> Bus Assignment2/1
  Vector Concatenate1/1 -> bytes/1
  Pack Spot Light Message8/2 -> Add2/9
  Pack Spot Light Message7/2 -> Add2/8
  Pack Spot Light Message6/2 -> Add2/7
  Pack Spot Light Message5/2 -> Add2/6
  Pack Spot Light Message4/2 -> Add2/5
  Pack Spot Light Message3/2 -> Add2/4
  Pack Spot Light Message2/2 -> Add2/3
  Pack Spot Light Message1/2 -> Add2/2
  Pack Spot Light Message/2 -> Add2/1

== matlab function ExampleWater/Pier/spotlight for each street light/MATLAB Function ==
  data: qb2n input; matCb2n output
function matCb2n = Cb2n(qb2n)
    q = [qb2n(1), qb2n(2), qb2n(3), qb2n(4)];
    matCb2n = quat2rotm(q);
end
